simulink model "Controller_MRC_Adaptive"  (R2019b)
settings: Solver=VariableStepAuto  StartTime=0.0  StopTime=500  RelTol=1e-3
libraries: slctrlblks x2
settings Model: Creator=Henry  LastModifiedBy=Kevin
settings SFSimCC: CustomCodeUndefinedFunction=UseInterfaceOnly

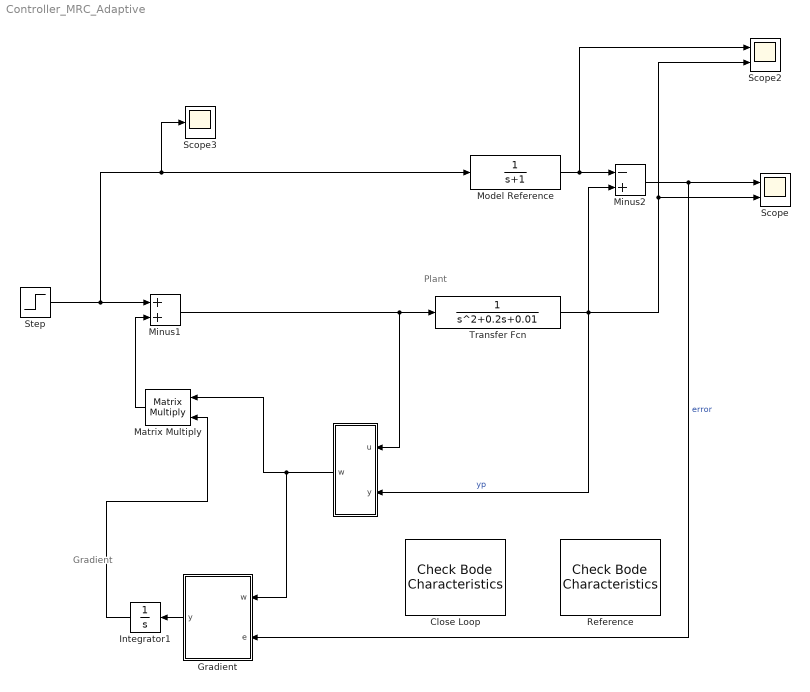
== system Controller_MRC_Adaptive ==
  note: Plant
  note: Gradient
  " " : Subsystem
  Close Loop : slctrlblks/Model Verification/Check Bode  Characteristics  InstantiateOnLoad=on  SaveOperatingPoints=off  LinearizationIOs={'/Transfer Fcn', 1, 'out', 'off', '';'/Minus1', 1, 'in', 'off', ''}  LinearizeAt=SnapshotTimes  SnapshotTimes=[0]  TriggerType=rising  SampleTime=auto  RateConversionMethod=zoh  PreWarpFreq=10  UseExactDelayModel=off  UseFullBlockNameLabels=off  UseBusSignalLabels=off  enabled=on  stopWhenAssertionFail=off  export=off  ViewDlgPos=[100 200 510 390]  OpenViewOnLoad=off  LaunchViewOnOpen=on  FrequencyUnits=rad/s  MagnitudeUnits=dB  PhaseUnits=deg  TimeUnits=seconds  EnableUpperBound=off  UpperBoundFrequencies=[]  UpperBoundMagnitudes=[]  EnableLowerBound=off  LowerBoundFrequencies=[]  LowerBoundMagnitudes=[]
      settings: SourceProductName=Simulink Control Design
  Gradient : MATLAB Function  TreatAsAtomicUnit=on
  Integrator1 : Integrator
  Matrix Multiply : Product  Multiplication=Matrix(*)
  Minus1 : Sum
  Minus2 : Sum  Inputs=-+
  Model Reference : TransferFcn  Denominator=[1 1]
  Reference : slctrlblks/Model Verification/Check Bode  Characteristics  InstantiateOnLoad=on  SaveOperatingPoints=off  LinearizationIOs={'/Model Reference', 1, 'out', 'off', '';'/Step', 1, 'in', 'off', ''}  LinearizeAt=SnapshotTimes  SnapshotTimes=[0]  TriggerType=rising  SampleTime=auto  RateConversionMethod=zoh  PreWarpFreq=10  UseExactDelayModel=off  UseFullBlockNameLabels=off  UseBusSignalLabels=off  enabled=on  stopWhenAssertionFail=off  export=off  ViewDlgPos=[100 200 510 390]  OpenViewOnLoad=off  LaunchViewOnOpen=on  FrequencyUnits=rad/s  MagnitudeUnits=dB  PhaseUnits=deg  TimeUnits=seconds  EnableUpperBound=off  UpperBoundFrequencies=[]  UpperBoundMagnitudes=[]  EnableLowerBound=off  LowerBoundFrequencies=[]  LowerBoundMagnitudes=[]
      settings: SourceProductName=Simulink Control Design
  Scope : Scope  NumInputPorts=2
  Scope2 : Scope  NumInputPorts=2
  Scope3 : Scope
  Step : Step  SampleTime=0
  Transfer Fcn : TransferFcn  Denominator=[1 ,0.2 ,0.01]
  wires:
  Model Reference/1 -> Scope2/1, Minus2/1
  Transfer Fcn/1 -> Scope2/2, Scope/2, " "/2("y "), Minus2/2  "yp"
  Step/1 -> Scope3/1, Model Reference/1, Minus1/1
  Minus1/1 -> " "/1("u "), Transfer Fcn/1
  Matrix Multiply/1 -> Minus1/2
  Gradient/1(y) -> Integrator1/1
  " "/1(w) -> Gradient/1(w), Matrix Multiply/1
  Minus2/1 -> Scope/1, Gradient/2(e)  "error"
  Integrator1/1 -> Matrix Multiply/2

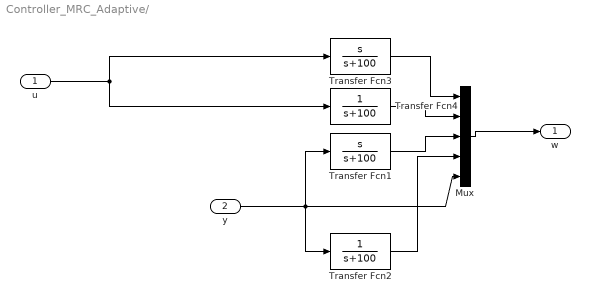
== system Controller_MRC_Adaptive/  ==
  "u " : Inport
  "y " : Inport  Port=2
  Mux : Mux  Inputs=5
  Transfer Fcn1 : TransferFcn  Numerator=[1 0]  Denominator=[1 100]
  Transfer Fcn2 : TransferFcn  Denominator=[1 100]
  Transfer Fcn3 : TransferFcn  Numerator=[1 0]  Denominator=[1 100]
  Transfer Fcn4 : TransferFcn  Denominator=[1 100]
  w : Outport
  wires:
  Transfer Fcn1/1 -> Mux/3
  "u "/1 -> Transfer Fcn3/1, Transfer Fcn4/1
  Mux/1 -> w/1
  "y "/1 -> Mux/5, Transfer Fcn2/1, Transfer Fcn1/1
  Transfer Fcn2/1 -> Mux/4
  Transfer Fcn3/1 -> Mux/1
  Transfer Fcn4/1 -> Mux/2

== matlab function Controller_MRC_Adaptive/Gradient ==
  data: w input; y output; e input
function y = fcn(w, e)
alpha = 0.01;
I = eye(5);
gamma = alpha*I;

%deadzone implementation
delta= 0.1;
if abs(e) > delta
    y = -gamma*w*e;
else
    y = 0;
end
